simulink subsystem "ComputeIfChanged"  (R2024a)
settings: Solver=VariableStepAuto  StartTime=0.0  StopTime=10.0  RelTol=1e-3
settings Model: Creator=dfurodet  LastModifiedBy=dfurodet

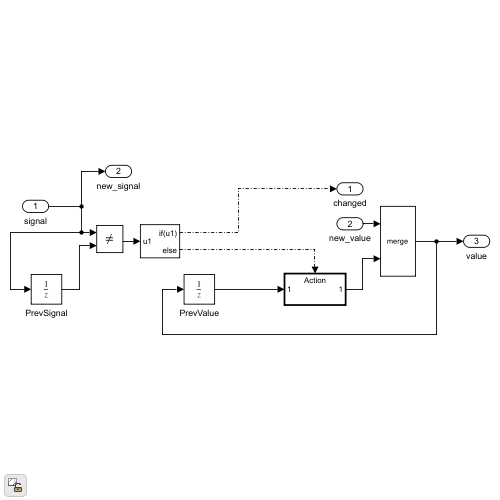
[thumbnail: Simulink's stored preview of the top-level diagram]
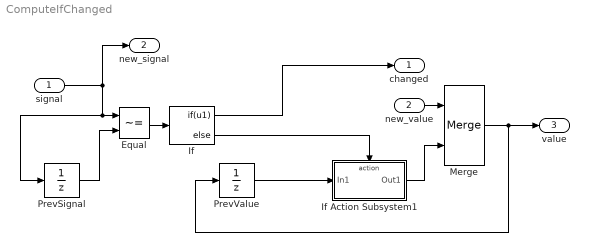
== system ComputeIfChanged ==
  signal : Inport
  new_value : Inport  Port=2
  Equal : RelationalOperator  Operator=~=  OutDataTypeStr=boolean  RndMeth=Simplest  InputSameDT=off
  If : If  IfExpression=u1
  If Action Subsystem1 : Subsystem  TreatAsAtomicUnit=on
  Merge : Merge
  PrevSignal : UnitDelay  SampleTime=-1  HasFrameUpgradeWarning=on
  PrevValue : UnitDelay  SampleTime=-1  HasFrameUpgradeWarning=on
  changed : Outport
  new_signal : Outport  Port=2
  value : Outport  Port=3
  wires:
  If/1 -> changed/1
  Equal/1 -> If/1
  signal/1 -> PrevSignal/1, Equal/1, new_signal/1
  Merge/1 -> PrevValue/1, value/1
  PrevValue/1 -> If Action Subsystem1/1(In1)
  If Action Subsystem1/1(Out1) -> Merge/2
  PrevSignal/1 -> Equal/2
  If/2 -> If Action Subsystem1/Action
  new_value/1 -> Merge/1

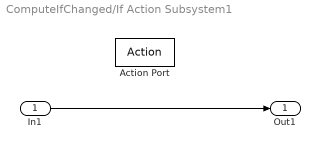
== system ComputeIfChanged/If Action Subsystem1 ==
  In1 : Inport
  Action Port : ActionPort
  Out1 : Outport
  wires:
  In1/1 -> Out1/1
